simulink model "ACC_speed_change_curve_cs"  (R2016a)
settings: Solver=ode5  SolverMode=SingleTasking  StartTime=0.0  StopTime=inf  FixedStep=1/1000  RelTol=1e-3
PreLoadFcn:
  | mbxruntime.callbacks.PreLoadFcn(bdroot);
  | check_NUTS_defined;
  | 
  | assignin('base',['model_closed_' bdroot],false);addpath('../includes_ACC');
PostLoadFcn:
  | mbxruntime.callbacks.PostLoadFcn(bdroot);
InitFcn:
  | mbxruntime.callbacks.InitFcn(bdroot);
StartFcn:
  | mbxruntime.callbacks.StartFcn(bdroot);
StopFcn:
  | mbxruntime.callbacks.StopFcn(bdroot);
model workspace (MAT data in the model file):
  mbox_table : struct (value not decoded)
  model_closed = 0
  sim_status = 0
undefined symbols (not defined in the file or in its folder): DiscIntNeverNeededParam
undefined symbols (not defined in the file): SteeringColumn, SteeringWheel, WheelL0, WheelL1, WheelR0, WheelR1
libraries: simulink_extras x49, simulink x29, PreScanSimulinkLibrary x24, PreScanUsefulBlocks x2, Solver_SF x1, simulink_need_slupdate x1
(part 2 of 17)

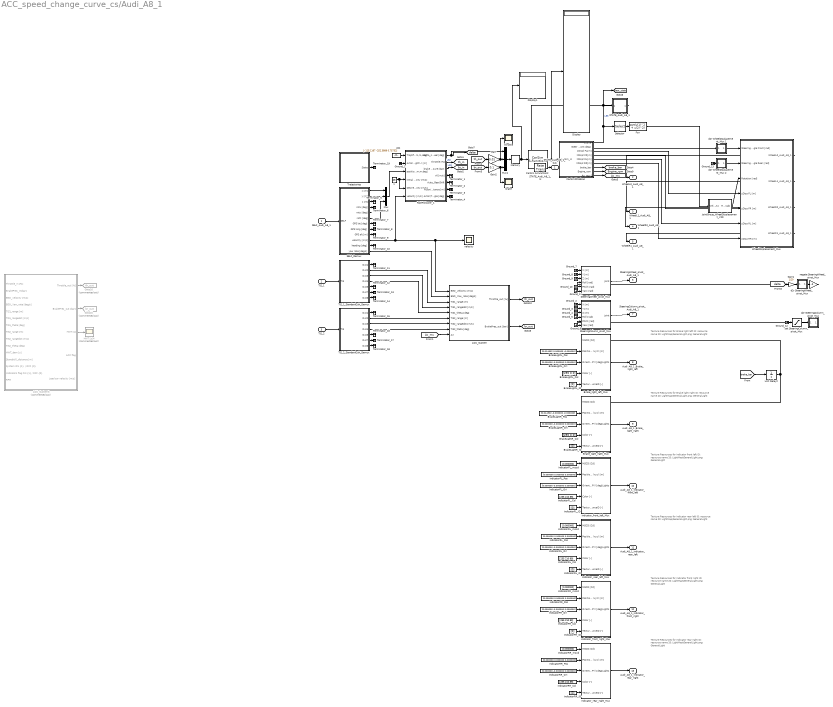
== system ACC_speed_change_curve_cs/Audi_A8_1 ==
  note: Texture Resources for Brake light left
      |
      | ID: resource name
      | 20: LightMap\GeneralLight.png: GeneralLight
  note: Texture Resources for Brake light right
      |
      | ID: resource name
      | 20: LightMap\GeneralLight.png: GeneralLight
  note: Texture Resources for Indicator front left
      |
      | ID: resource name
      | 20: LightMap\GeneralLight.png: GeneralLight
  note: Texture Resources for Indicator rear left
      |
      | ID: resource name
      | 20: LightMap\GeneralLight.png: GeneralLight
  note: Texture Resources for Indicator front right
      |
      | ID: resource name
      | 20: LightMap\GeneralLight.png: GeneralLight
  note: Texture Resources for Indicator rear right
      |
      | ID: resource name
      | 20: LightMap\GeneralLight.png: GeneralLight
  SELF_Audi_A8_1 : Inport  Tag=inport/SelfPort  OutDataTypeStr=Bus: PRESCAN_SELFSENSORDATA  PortDimensions=1  SampleTime=20/1000  BusOutputAsStruct=on
  TIS_1 : Inport  Tag=inport/TIS  Port=2  OutDataTypeStr=Bus: PRESCAN_SCANNERSENSOR_MESSAGE  PortDimensions=32  SampleTime=1/25  BusOutputAsStruct=on
  TIS_2 : Inport  Tag=inport/TIS  Port=3  OutDataTypeStr=Bus: PRESCAN_SCANNERSENSOR_MESSAGE  PortDimensions=32  SampleTime=1/25  BusOutputAsStruct=on
  ACC_System : Subsystem  mask(ACC System){J_xx=210, Rw=0.34, LaneWidth=3.5, Qfac=40.4695, BrakePressureMax=150, BrakeMax=3.5, MaxSpeed=200, drd=3, LowSpeedActv=40, TISMaxRange=[150 30], TISMaxTheta=[9 80], Tblock=1/100, TISsensor=[1/25 1/25], TISdet=[32 32], DisplaySwitch=on, DisplayFreq=25, RadarSwitch=on, RadarFreq=25}
      mask prompts: J_xx "Principal moment of inertia along longitudal (x) axis Jxx [kg*m^2]"; Rw "Tyre radius Rw [m]"; LaneWidth "Width of the lane [m]"; Qfac "Conversion factor of braking pressure into braking torque Qfac [Nm/bar]"; BrakePressureMax "Maximum brake pressure (that the controller can apply) [bar]"; BrakeMax "Maximum acceleration / deceleration, which can be applied by ACC [m/s^2]"; MaxSpeed "Maximum ACC operating velocity [km/h]"; drd "Cut-Off relatve velocity of EGO and LEAD [km/h]"; LowSpeedActv "LEAD Cut-Off Speed [km/h]"; TISMaxRange "TIS maximum range (TIS1 and TIS2) [m]"; TISMaxTheta "TIS maximum theta angle (TIS1 and TIS2) [deg]"; Tblock "Target update rate of the compilation sheet [s]"; TISsensor "TIS update rate (TIS1 and TIS2) [s]"; TISdet "TIS max. objects to detect (TIS1 and TIS2)"; DisplaySwitch "Show EGO parameters visualization"; DisplayFreq "EGO parameters visualization frequency [Hz]"; RadarSwitch "Show radar visualization"; RadarFreq "Radar frequency [Hz]"
      mask help: PreScan Experiment and Simple Dynamics model parameters
      mask init:
      | Tsensor = max([TISsensor]);
      mask Help: eval('openHelp(1131)')
      mask Callback DisplaySwitch:
      | en = get_param(gcb,'MaskEnables');
      | switch get_param(gcb, 'DisplaySwitch')
      |     case 'off'
      |         en{16} = 'off';
      |     case 'on'
      |         en{16} = 'on';
      | end
      | set_param(gcb,'MaskEnables',en);
      | clear en;
      mask Callback RadarSwitch:
      | en = get_param(gcb,'MaskEnables');
      | switch get_param(gcb, 'RadarSwitch')
      |     case 'off'
      |         en{18} = 'off';
      |     case 'on'
      |         en{18} = 'on';
      | end
      | set_param(gcb,'MaskEnables',en);
      | clear en;
  ACC_System3 : Subsystem  Commented=on  mask(ACC System){J_xx=210, Rw=0.34, LaneWidth=3.5, Qfac=40.4695, BrakePressureMax=150, MaxSpeed=200, drd=3, LowSpeedActv=40, TISMaxRange=[150 30], TISMaxTheta=[9 80], Tblock=1/100, TISsensor=[1/25 1/25], TISdet=[32 32], DisplaySwitch=on, DisplayFreq=25, RadarSwitch=on, RadarFreq=25, BrakeMax=10, BrakeRateMax=100, b=0.1, p=1, i=0.2, d=0}
      mask prompts: J_xx "Principal moment of inertia along longitudal (x) axis Jxx [kg*m^2]"; Rw "Tyre radius Rw [m]"; LaneWidth "Width of the lane [m]"; Qfac "Conversion factor of braking pressure into braking torque Qfac [Nm/bar]"; BrakePressureMax "Maximum brake pressure (that the controller can apply) [bar]"; MaxSpeed "Maximum ACC operating velocity [km/h]"; drd "Cut-Off relatve velocity of EGO and LEAD [km/h]"; LowSpeedActv "LEAD Cut-Off Speed [km/h]"; TISMaxRange "TIS maximum range (TIS1 and TIS2) [m]"; TISMaxTheta "TIS maximum theta angle (TIS1 and TIS2) [deg]"; Tblock "Target update rate of the compilation sheet [s]"; TISsensor "TIS update rate (TIS1 and TIS2) [s]"; TISdet "TIS max. objects to detect (TIS1 and TIS2)"; DisplaySwitch "Show EGO parameters visualization"; DisplayFreq "EGO parameters visualization frequency [Hz]"; RadarSwitch "Show radar visualization"; RadarFreq "Radar frequency [Hz]"; BrakeMax "Maximum acceleration / deceleration, which can be applied by ACC [m/s^2]"; BrakeRateMax "Maximum acceleration/deceleration change rate"; b "brake gain"; p "throttle p"; i "throttle i"; d "throttle d"
      mask help: PreScan Experiment and Simple Dynamics model parameters
      mask init:
      | Tsensor = max([TISsensor]);
      mask Help: eval('openHelp(1131)')
      mask Callback DisplaySwitch:
      | en = get_param(gcb,'MaskEnables');
      | switch get_param(gcb, 'DisplaySwitch')
      |     case 'off'
      |         en{16} = 'off';
      |     case 'on'
      |         en{16} = 'on';
      | end
      | set_param(gcb,'MaskEnables',en);
      | clear en;
      mask Callback RadarSwitch:
      | en = get_param(gcb,'MaskEnables');
      | switch get_param(gcb, 'RadarSwitch')
      |     case 'off'
      |         en{18} = 'off';
      |     case 'on'
      |         en{18} = 'on';
      | end
      | set_param(gcb,'MaskEnables',en);
      | clear en;
  BrakeLightL_Col : Constant  Tag=VisuLightConst  Value=[255 0 0]
  BrakeLightL_ID : Constant  Tag=VisuLightConst  Value=[0]
  BrakeLightL_Ori : Constant  Tag=VisuLightConst  Value=[0.000000 -0.000000 0.000000]
  BrakeLightL_Pos : Constant  Tag=VisuLightConst  Value=[0.014502 0.000000 -0.000000]
  BrakeLightR_Col : Constant  Tag=VisuLightConst  Value=[255 0 0]
  BrakeLightR_ID : Constant  Tag=VisuLightConst  Value=[0]
  BrakeLightR_Ori : Constant  Tag=VisuLightConst  Value=[0.000000 -0.000000 0.000000]
  BrakeLightR_Pos : Constant  Tag=VisuLightConst  Value=[0.014502 -0.000000 -0.000000]
  Brake_light_left_Mux : Subsystem  Tag=mux/ActiveLight  mask(PreScan User Interface: VisuActiveLight){}
      mask help:
      | The VisuActiveLight block provides a way for detailed animation of Light Sources, such as the indicator, brake, fog and main lights of a vehicle, or a light post.
      |
      | For more information, please click Help.
      settings: DeleteFcn=PreScanBlockDeleteFcn;
      mask Help: eval('openHelp(209)')
  Brake_light_right_Mux : Subsystem  Tag=mux/ActiveLight  mask(PreScan User Interface: VisuActiveLight){}
      mask help:
      | The VisuActiveLight block provides a way for detailed animation of Light Sources, such as the indicator, brake, fog and main lights of a vehicle, or a light post.
      |
      | For more information, please click Help.
      settings: DeleteFcn=PreScanBlockDeleteFcn;
      mask Help: eval('openHelp(209)')
  CarSim S-Function2 : Solver_SF/CarSim S-Function2  Priority=1  VehicleCode=i_i  SIMFILE=C:\Users\Public\Documents\CarSim2016Data\simfile.sim
      settings: AttributesFormatString=Vehicle Code: %<VehicleCode>
  CarSim2PreScan : Subsystem  mask(CarSim2PreScan:){z0=0, z0_ini_VRML=0.3}
      mask prompts: z0 "PreScan Actor initial COG z-position wrt GLOBAL axis system [m]"; z0_ini_VRML "z_ini_VRML [m]. Taken from : "VISUWheels_<ActorName>/conv_TransWheel.../pos_ini_Visu/z_ini_VRML" block. Use a Display Simulink block in order to visualize the value."
      mask help: This block converts the outputs coming from the CarSim block into consistent PreScan signals.
  Display : Display
  Display1 : Display
  Fcn : Fcn  Expr=sqrt(u(1)^2 + u(2)^2)
  Gain : Gain  Gain=0.01
  Gain1 : Gain  Gain=1/20
  Gain2 : Gain  Gain=0.1
  Goto15 : Goto  Commented=on  GotoTag=br_out  TagVisibility=global
  Goto16 : Goto  Commented=on  GotoTag=th_out  TagVisibility=global
  Ground_{1..13} (13 alike) : Ground
  HWT [s]4 : Scope  Commented=on
  IndicatorFL_Col : Constant  Tag=VisuLightConst  Value=[255 210 89]
  IndicatorFL_ID : Constant  Tag=VisuLightConst  Value=[0]
  IndicatorFL_Ori : Constant  Tag=VisuLightConst  Value=[0.000000 -0.000000 0.000000]
  IndicatorFL_Pos : Constant  Tag=VisuLightConst  Value=[0.000000 0.000000 0.000000]
  IndicatorFL_mscd : Constant  Tag=VisuLightConst  Value=[0.000000]
  IndicatorFR_Col : Constant  Tag=VisuLightConst  Value=[255 210 89]
  IndicatorFR_ID : Constant  Tag=VisuLightConst  Value=[0]
  IndicatorFR_Ori : Constant  Tag=VisuLightConst  Value=[0.000000 -0.000000 0.000000]
  IndicatorFR_Pos : Constant  Tag=VisuLightConst  Value=[0.000000 0.000000 0.000000]
  IndicatorFR_mscd : Constant  Tag=VisuLightConst  Value=[0.000000]
  IndicatorRL_Col : Constant  Tag=VisuLightConst  Value=[255 210 89]
  IndicatorRL_ID : Constant  Tag=VisuLightConst  Value=[0]
  IndicatorRL_Ori : Constant  Tag=VisuLightConst  Value=[0.000000 -0.000000 0.000000]
  IndicatorRL_Pos : Constant  Tag=VisuLightConst  Value=[0.000000 0.000000 0.000000]
  IndicatorRL_mscd : Constant  Tag=VisuLightConst  Value=[0.000000]
  IndicatorRR_Col : Constant  Tag=VisuLightConst  Value=[255 210 89]
  IndicatorRR_ID : Constant  Tag=VisuLightConst  Value=[0]
  IndicatorRR_Ori : Constant  Tag=VisuLightConst  Value=[0.000000 -0.000000 0.000000]
  IndicatorRR_Pos : Constant  Tag=VisuLightConst  Value=[0.000000 0.000000 0.000000]
  IndicatorRR_mscd : Constant  Tag=VisuLightConst  Value=[0.000000]
  Indicator_front_left_Mux : Subsystem  Tag=mux/ActiveLight  mask(PreScan User Interface: VisuActiveLight){}
      mask help:
      | The VisuActiveLight block provides a way for detailed animation of Light Sources, such as the indicator, brake, fog and main lights of a vehicle, or a light post.
      |
      | For more information, please click Help.
      settings: DeleteFcn=PreScanBlockDeleteFcn;
      mask Help: eval('openHelp(209)')
  Indicator_front_right_Mux : Subsystem  Tag=mux/ActiveLight  mask(PreScan User Interface: VisuActiveLight){}
      mask help:
      | The VisuActiveLight block provides a way for detailed animation of Light Sources, such as the indicator, brake, fog and main lights of a vehicle, or a light post.
      |
      | For more information, please click Help.
      settings: DeleteFcn=PreScanBlockDeleteFcn;
      mask Help: eval('openHelp(209)')
  Indicator_rear_left_Mux : Subsystem  Tag=mux/ActiveLight  mask(PreScan User Interface: VisuActiveLight){}
      mask help:
      | The VisuActiveLight block provides a way for detailed animation of Light Sources, such as the indicator, brake, fog and main lights of a vehicle, or a light post.
      |
      | For more information, please click Help.
      settings: DeleteFcn=PreScanBlockDeleteFcn;
      mask Help: eval('openHelp(209)')
  Indicator_rear_right_Mux : Subsystem  Tag=mux/ActiveLight  mask(PreScan User Interface: VisuActiveLight){}
      mask help:
      | The VisuActiveLight block provides a way for detailed animation of Light Sources, such as the indicator, brake, fog and main lights of a vehicle, or a light post.
      |
      | For more information, please click Help.
      settings: DeleteFcn=PreScanBlockDeleteFcn;
      mask Help: eval('openHelp(209)')
  JointGroup_WheelDisplacement_V2R : Subsystem  Tag=mux/Wheels  mask(PreScan Velocity to Wheel Angle Block:){TimeStep=20/1000, TireRadius=0.34000000357627869}
      mask prompts: TimeStep "Auto Assigned: Time Step [s]"; TireRadius "Tire Radius [m]"
      settings: DeleteFcn=PreScanBlockDeleteFcn;
      mask Display: disp('Velocity\nto\nWheelAngle')
  Memory : Memory
  Mux : Mux  Inputs=3
  Mux1 : Mux  Inputs=3
  PathFollower_1 : Subsystem  Tag=pathFollower  mask(PreScan Block: Path Follower){Migrate=on, FileName='Trajectory_1.mat', TunableSteeringGain=1, XShifting_wrt_COG=0}
      mask prompts: Migrate "Migrate. During migration this block will be replaced by a newer one."; FileName "Trajectory Name"; TunableSteeringGain "TunableSteeringGain [-]"; XShifting_wrt_COG "XShifting_wrt_COG [m]"
      mask help:
      | The Path Follower Model is selected in the GUI to simulate driver behavior.
      |
      | For more information, please click Help.
      mask init:
      | load(['trajectories/',eval(FileName)])
      | traject=trajectory';
      | 
      | Traj_x=traject(:,2);
      | Traj_y=traject(:,3);
      | Traj_z=traject(:,4);
      | Traj_vx=traject(:,8);
      | Traj_vy=traject(:,9);
      | Traj_vz=traject(:,10);
      mask Help: eval('openHelp(232)')
  SELF_Demux : Subsystem  Tag=demux/SelfPort  mask(PreScan Demux Block:){}
      mask help:
      | The SELF port shows (state) information of the actor itself. The outputs are position in the experiment's axis system and the GPS coordinates, and the object's absolute velocity and compass heading.
      |
      | For more information, please click Help.
      settings: DeleteFcn=PreScanBlockDeleteFcn;
      mask Help: eval('openHelp(462)')
      mask Display:
      | port_label('output',1,'x [m]')
      | port_label('output',2,'y [m]')
      | port_label('output',3,'z [m]','texmode','on')
      | port_label('output',4,'Rotx [deg]','texmode','on')
      | port_label('output',5,'Roty [deg]','texmode','on')
      | port_label('output',6,'Rotz [deg]','texmode','on')
      | port_label('output',7,'GPS lat [deg]','texmode','on')
      | port_label('output',8,'GPS long [deg]','texmode','on')
      | port_label('output',9,'GPS alt [m]','texmode','on')
      | port_label('output',10,'Velocity [m/s]')
      | port_label('output',11,'Heading [deg]')
      | port_label('output',12,'Yaw rate [deg/s]')
  STATE_Audi_A8_1 : Subsystem  Tag=mux/StatePort  Priority=0  LoadFcn=load PrescanStateActuatorData  mask(PreScan Sink Block: State){x0=-115.1167, y0=-252.3889, z0=0.55, Roll0=0, Pitch0=0, Yaw0=0.75732, TimeStep=20/1000}
      mask prompts: x0 "Ini x-position VEHICLE wrt GLOBAL axis system [m]"; y0 "Ini y-position VEHICLE wrt GLOBAL axis system [m]"; z0 "Ini z-position VEHICLE wrt GLOBAL axis system [m]"; Roll0 "Ini roll-angle BODY wrt VEHICLE axis system [deg]"; Pitch0 "Ini pitch-angle BODY wrt VEHICLE axis system [deg]"; Yaw0 "Ini yaw-angle VEHICLE wrt GLOBAL axis system [deg]"; TimeStep "Auto-Assigned: Upload Period [s]"
      mask help:
      | The Actor State contains a vector signal of size (9x1), containing the following signals:
      |
      | -  Position                  (x,y,z)                                     [m]
      | -  Velocity                  (vx,vy,vz)                               [m/s]
      | -  Angles                    (Roll, Pitch, Yaw)                   [rad]
      |
      | The Actor state is defined in the global axis system.
      | The state is superponed on the Initial position defined in the GUI.
      |
      | For more information, please click Help.
      settings: DeleteFcn=PreScanBlockDeleteFcn;
      mask Help: eval('openHelp(222)')
      mask Display: image(imread('State.png'))
  STATE_Audi_A8_1_rc : RateTransition  Tag=mux_rc/StatePort  OutPortSampleTimeOpt=Inherit
  Selector : Selector  InputPortWidth=9  IndexOptions=Index vector (dialog)  Indices=[4 5]  OutputSizes=1
  SteeringColumn_pivot_Mux : Subsystem  Tag=mux/Joint  mask(PreScan Mux Block){DisplayName=SteeringColumn}
      mask prompts: DisplayName "Display Name"
      mask help:
      | This block simulates a generic joint used for generic models. This joint can be enabled/disabled from the GUI.
      |
      | For more information, please click Help.
      settings: DeleteFcn=PreScanBlockDeleteFcn;
      mask Help: eval('openHelp(254)')
  SteeringWheel_pivot_Mux : Subsystem  Tag=mux/Joint  mask(PreScan Mux Block){DisplayName=SteeringWheel}
      mask prompts: DisplayName "Display Name"
      mask help:
      | This block simulates a generic joint used for generic models. This joint can be enabled/disabled from the GUI.
      |
      | For more information, please click Help.
      settings: DeleteFcn=PreScanBlockDeleteFcn;
      mask Help: eval('openHelp(254)')
  TIS_1_StandardCoh_Demux : Subsystem  Tag=demux/TIS/StandardCoh  TreatAsAtomicUnit=on  mask(PreScan Demux Block: TIS){MAXMESSAGES=32}
      mask prompts: MAXMESSAGES "Number of Objects"
      mask Help: eval('openHelp(449)')
      mask Display:
      | port_label('input',1,'TIS')
      | port_label('output',1,'Beam ID [-]')
      | port_label('output',2,'Range [m]')
      | port_label('output',3,'DopplerVelocity [m/s]')
      | port_label('output',4,'{\theta} [deg]','texmode','on')
      | port_label('output',5,'{\phi} [deg]','texmode','on')
      | port_label('output',6,'Target ID [-]','texmode','on')
      | port_label('output',7,'TIS Data','texmode','on')
  TIS_2_StandardCoh_Demux : Subsystem  Tag=demux/TIS/StandardCoh  TreatAsAtomicUnit=on  mask(PreScan Demux Block: TIS){MAXMESSAGES=32}
      mask prompts: MAXMESSAGES "Number of Objects"
      mask Help: eval('openHelp(449)')
      mask Display:
      | port_label('input',1,'TIS')
      | port_label('output',1,'Beam ID [-]')
      | port_label('output',2,'Range [m]')
      | port_label('output',3,'DopplerVelocity [m/s]')
      | port_label('output',4,'{\theta} [deg]','texmode','on')
      | port_label('output',5,'{\phi} [deg]','texmode','on')
      | port_label('output',6,'Target ID [-]','texmode','on')
      | port_label('output',7,'TIS Data','texmode','on')
  Terminator_{1..19} (19 alike) : Terminator
  Trajectories : Subsystem  Tag=Trajectories  mask(PreScan Source Block: Trajectories){}
      mask help:
      | The Trajectory block contains the trajectories defined in the PreScan Experiment Editor. The output of the trajectory block is the (vehicle) State.
      |
      | For more information, please click Help.
      settings: DeleteFcn=PreScanBlockDeleteFcn;
      mask Help: eval('openHelp(312)')
      mask Display: image(imread('Trajectory.png'));
  Unit Delay2 : UnitDelay  InitialCondition=1  SampleTime=-1
  V : Constant  Value=28
  WheelDisplacement_Mux : Subsystem  Tag=mux/JointGroup  mask(JointGroup){}
      mask help:
      | The JointGroup allows to control several Joints in one go, as defined for this particular model.
      | For more information, look in the PreScan manual in the section "Model Preparation Tool" -> "Joint Groups"
      |
      | For more information on the Joints simulink interface, press Help.
      mask Help: eval('openHelp(254)')
  brake : Scope
  d2r SteeringColumn_pivot_Mux : Subsystem  mask(DegreesToRadians){}
      mask help: SimulinkBlocks:simulink_extras:DegreesToRadians_MD
      mask Help: web([docroot '/simulink/ref_extras/degreestoradians.html'])
      mask Display: disp('D2R')
  d2r SteeringWheel_pivot_Mux : Subsystem  mask(DegreesToRadians){}
      mask help: SimulinkBlocks:simulink_extras:DegreesToRadians_MD
      mask Help: web([docroot '/simulink/ref_extras/degreestoradians.html'])
      mask Display: disp('D2R')
  d2r WheelDisplacement_Mux 1 : Subsystem  mask(DegreesToRadians){}
      mask help: SimulinkBlocks:simulink_extras:DegreesToRadians_MD
      mask Help: web([docroot '/simulink/ref_extras/degreestoradians.html'])
      mask Display: disp('D2R')
  d2r WheelDisplacement_Mux 2 : Subsystem  mask(DegreesToRadians){}
      mask help: SimulinkBlocks:simulink_extras:DegreesToRadians_MD
      mask Help: web([docroot '/simulink/ref_extras/degreestoradians.html'])
      mask Display: disp('D2R')
  negate SteeringWheel_pivot_Mux : Gain  Gain=-1
  pos : Constant  Tag=pos  Value=[-115.1167 -252.3889 0.75732]
  sat SteeringColumn_pivot_Mux : Saturate  UpperLimit=30  LowerLimit=-5
  throttle : Scope
  "velocity " : Scope
  STATE_Audi_A8_1_bus : Outport  Tag=outport/StatePort  OutDataTypeStr=Bus: PRESCAN_STATEACTUATORDATA  PortDimensions=1  SampleTime=20/1000
  WheelL0_Audi_A8_1 : Outport  Tag=outport/JointActuator  Port=2  OutDataTypeStr=Bus: PRESCAN_POSE_DATA  SampleTime=20/1000
  WheelL1_Audi_A8_1 : Outport  Tag=outport/JointActuator  Port=3  OutDataTypeStr=Bus: PRESCAN_POSE_DATA  SampleTime=20/1000
  WheelR0_Audi_A8_1 : Outport  Tag=outport/JointActuator  Port=4  OutDataTypeStr=Bus: PRESCAN_POSE_DATA  SampleTime=20/1000
  WheelR1_Audi_A8_1 : Outport  Tag=outport/JointActuator  Port=5  OutDataTypeStr=Bus: PRESCAN_POSE_DATA  SampleTime=20/1000
  SteeringWheel_pivot_Audi_A8_1 : Outport  Tag=outport/JointActuator  Port=6  OutDataTypeStr=Bus: PRESCAN_POSE_DATA  SampleTime=20/1000
  SteeringColumn_pivot_Audi_A8_1 : Outport  Tag=outport/JointActuator  Port=7  OutDataTypeStr=Bus: PRESCAN_POSE_DATA  SampleTime=20/1000
  Audi_A8_1_Brake_light_left : Outport  Tag=outport/BrakeLightL  Port=8  OutDataTypeStr=Bus: PRESCAN_VISULIGHTACTUATOR_DATA  SampleTime=20/1000
  Audi_A8_1_Brake_light_right : Outport  Tag=outport/BrakeLightR  Port=9  OutDataTypeStr=Bus: PRESCAN_VISULIGHTACTUATOR_DATA  SampleTime=20/1000
  Audi_A8_1_Indicator_front_left : Outport  Tag=outport/IndicatorFL  Port=10  OutDataTypeStr=Bus: PRESCAN_VISULIGHTACTUATOR_DATA  SampleTime=20/1000
  Audi_A8_1_Indicator_rear_left : Outport  Tag=outport/IndicatorRL  Port=11  OutDataTypeStr=Bus: PRESCAN_VISULIGHTACTUATOR_DATA  SampleTime=20/1000
  Audi_A8_1_Indicator_front_right : Outport  Tag=outport/IndicatorFR  Port=12  OutDataTypeStr=Bus: PRESCAN_VISULIGHTACTUATOR_DATA  SampleTime=20/1000
  Audi_A8_1_Indicator_rear_right : Outport  Tag=outport/IndicatorRR  Port=13  OutDataTypeStr=Bus: PRESCAN_VISULIGHTACTUATOR_DATA  SampleTime=20/1000
  tag scope: Ax_ms=global, Engine_rpm=global, br_in=global, br_out=global, brake_bar=global, delta=global, th_in=global, th_out=global, view_state=global
  wires:
  sat SteeringColumn_pivot_Mux/1 -> d2r SteeringColumn_pivot_Mux/1(Degrees in)
  d2r SteeringColumn_pivot_Mux/1(Radians out) -> SteeringColumn_pivot_Mux/5(Pitch [rad])
  negate SteeringWheel_pivot_Mux/1 -> SteeringWheel_pivot_Mux/4(Roll [rad])
  d2r SteeringWheel_pivot_Mux/1(Radians out) -> negate SteeringWheel_pivot_Mux/1
  [brake_bar] -> Unit Delay2/1
  Unit Delay2/1 -> Brake_light_left_Mux/1(MSCD [Cd]), Brake_light_right_Mux/1(MSCD [Cd])
  [delta] -> Gain1/1
  Gain1/1 -> d2r SteeringWheel_pivot_Mux/1(Degrees in)
  PathFollower_1/2(throttle [%]) -> [th_in]  "L82"
  PathFollower_1/3(brake pressure [bar]) -> [br_in]  "L83"
  SELF_Demux/5(roty [deg]) -> ?
  Mux/1 -> PathFollower_1/3(position x,y,Y [m,m,deg])
  SELF_Demux/1(x [m]) -> Mux/1
  SELF_Demux/2(y [m]) -> Mux/2
  SELF_Demux/6(rotz [deg]) -> Mux/3
  V/1 -> PathFollower_1/4(Initial Velocity [m/s]), PathFollower_1/5(Desired Velocity [m/s])
  d2r WheelDisplacement_Mux 1/1(Radians out) -> WheelDisplacement_Mux/1(Steering Angle Front [rad])
  d2r WheelDisplacement_Mux 2/1(Radians out) -> WheelDisplacement_Mux/2(Steering Angle Rear [rad])
  CarSim2PreScan/3(zDispl FL[m]) -> WheelDisplacement_Mux/4(zDisp FL [m])
  CarSim2PreScan/4(zDispl FR[m]) -> WheelDisplacement_Mux/5(zDisp FR [m])
  CarSim2PreScan/5(zDispl RL[m]) -> WheelDisplacement_Mux/6(zDisp RL [m])
  CarSim2PreScan/6(zDispl RR[m]) -> WheelDisplacement_Mux/7(zDisp RR [m])
  CarSim2PreScan/2(Steer Angle Front [deg]) -> d2r WheelDisplacement_Mux 1/1(Degrees in)
  CarSim2PreScan/1(STATE) -> [view_state], STATE_Audi_A8_1/1(State), Selector/1  "L86"
  Fcn/1 -> JointGroup_WheelDisplacement_V2R/1(Velocity [m/s])
  Mux1/1 -> Memory/1
  CarSim S-Function2/1 -> Display/1, CarSim2PreScan/1(CarSim_In)
  Selector/1 -> Fcn/1
  CarSim2PreScan/7(brake_bar) -> [brake_bar]
  CarSim2PreScan/8(Engine_rpm) -> [Engine_rpm]
  Memory/1 -> Display1/1, CarSim S-Function2/1
  PathFollower_1/1(delta_steerwheel [deg]) -> Mux1/1, [delta]
  [th_out] -> Gain/1
  [br_out] -> Gain2/1
  Ground_13/1 -> d2r WheelDisplacement_Mux 2/1(Degrees in)
  TIS_2_StandardCoh_Demux/3(Out3) -> ACC_System/7(TIS2_rangedot [m/s])
  SELF_Demux/12(yaw rate [deg/s]) -> ACC_System/2(EGO_Yaw_rate [deg/s])
  TIS_1_StandardCoh_Demux/2(Out2) -> ACC_System/3(TIS1_range [m])
  TIS_1_StandardCoh_Demux/3(Out3) -> ACC_System/4(TIS1_rangedot [m/s])
  TIS_1_StandardCoh_Demux/4(Out4) -> ACC_System/5(TIS1_theta [deg])
  TIS_2_StandardCoh_Demux/2(Out2) -> ACC_System/6(TIS2_range [m])
  TIS_2_StandardCoh_Demux/4(Out4) -> ACC_System/8(TIS2_theta [deg])
  SELF_Demux/10(velocity [m/s]) -> ACC_System/1(EGO_velocity [m/s]), "velocity "/1, PathFollower_1/6(velocity [m/s])
  CarSim2PreScan/9(Ax_ms-1) -> [Ax_ms]
  Gain/1 -> throttle/1, Mux1/2
  Gain2/1 -> brake/1, Mux1/3
  ACC_System3/1(Throttle_out [%]) -> Goto16/1
  ACC_System3/2(BrakePres_out [bar]) -> Goto15/1
  ACC_System3/3(HWT [s]) -> HWT [s]4/1
  ACC_System/1(Throttle_out [%]) -> [th_out]
  ACC_System/2(BrakePres_out [bar]) -> [br_out]
  [Ax_ms] -> ACC_System/9(AX)
  STATE_Audi_A8_1_rc/1 -> STATE_Audi_A8_1_bus/1
  STATE_Audi_A8_1/1(StateBus) -> STATE_Audi_A8_1_rc/1
  SELF_Audi_A8_1/1 -> SELF_Demux/1(SELF)
  TIS_1/1 -> TIS_1_StandardCoh_Demux/1(TIS)
  TIS_2/1 -> TIS_2_StandardCoh_Demux/1(TIS)
  WheelDisplacement_Mux/1(WheelL0_Audi_A8_1) -> WheelL0_Audi_A8_1/1
  WheelDisplacement_Mux/2(WheelL1_Audi_A8_1) -> WheelL1_Audi_A8_1/1
  WheelDisplacement_Mux/3(WheelR0_Audi_A8_1) -> WheelR0_Audi_A8_1/1
  WheelDisplacement_Mux/4(WheelR1_Audi_A8_1) -> WheelR1_Audi_A8_1/1
  JointGroup_WheelDisplacement_V2R/1(Rotation [rad]) -> WheelDisplacement_Mux/3(Rotation [rad])
  SteeringWheel_pivot_Mux/1(Joint) -> SteeringWheel_pivot_Audi_A8_1/1
  SteeringColumn_pivot_Mux/1(Joint) -> SteeringColumn_pivot_Audi_A8_1/1
  Brake_light_left_Mux/1(Lights) -> Audi_A8_1_Brake_light_left/1
  BrakeLightL_Pos/1 -> Brake_light_left_Mux/2(Position (xyz) [m])
  BrakeLightL_Ori/1 -> Brake_light_left_Mux/3(Orientation (RPY) [deg])
  BrakeLightL_Col/1 -> Brake_light_left_Mux/4(Color [-])
  BrakeLightL_ID/1 -> Brake_light_left_Mux/5(TextureResourceID [-])
  Brake_light_right_Mux/1(Lights) -> Audi_A8_1_Brake_light_right/1
  BrakeLightR_Pos/1 -> Brake_light_right_Mux/2(Position (xyz) [m])
  BrakeLightR_Ori/1 -> Brake_light_right_Mux/3(Orientation (RPY) [deg])
  BrakeLightR_Col/1 -> Brake_light_right_Mux/4(Color [-])
  BrakeLightR_ID/1 -> Brake_light_right_Mux/5(TextureResourceID [-])
  Indicator_front_left_Mux/1(Lights) -> Audi_A8_1_Indicator_front_left/1
  IndicatorFL_mscd/1 -> Indicator_front_left_Mux/1(MSCD [Cd])
  IndicatorFL_Pos/1 -> Indicator_front_left_Mux/2(Position (xyz) [m])
  IndicatorFL_Ori/1 -> Indicator_front_left_Mux/3(Orientation (RPY) [deg])
  IndicatorFL_Col/1 -> Indicator_front_left_Mux/4(Color [-])
  IndicatorFL_ID/1 -> Indicator_front_left_Mux/5(TextureResourceID [-])
  Indicator_rear_left_Mux/1(Lights) -> Audi_A8_1_Indicator_rear_left/1
  IndicatorRL_mscd/1 -> Indicator_rear_left_Mux/1(MSCD [Cd])
  IndicatorRL_Pos/1 -> Indicator_rear_left_Mux/2(Position (xyz) [m])
  IndicatorRL_Ori/1 -> Indicator_rear_left_Mux/3(Orientation (RPY) [deg])
  IndicatorRL_Col/1 -> Indicator_rear_left_Mux/4(Color [-])
  IndicatorRL_ID/1 -> Indicator_rear_left_Mux/5(TextureResourceID [-])
  Indicator_front_right_Mux/1(Lights) -> Audi_A8_1_Indicator_front_right/1
  IndicatorFR_mscd/1 -> Indicator_front_right_Mux/1(MSCD [Cd])
  IndicatorFR_Pos/1 -> Indicator_front_right_Mux/2(Position (xyz) [m])
  IndicatorFR_Ori/1 -> Indicator_front_right_Mux/3(Orientation (RPY) [deg])
  IndicatorFR_Col/1 -> Indicator_front_right_Mux/4(Color [-])
  IndicatorFR_ID/1 -> Indicator_front_right_Mux/5(TextureResourceID [-])
  Indicator_rear_right_Mux/1(Lights) -> Audi_A8_1_Indicator_rear_right/1
  IndicatorRR_mscd/1 -> Indicator_rear_right_Mux/1(MSCD [Cd])
  IndicatorRR_Pos/1 -> Indicator_rear_right_Mux/2(Position (xyz) [m])
  IndicatorRR_Ori/1 -> Indicator_rear_right_Mux/3(Orientation (RPY) [deg])
  IndicatorRR_Col/1 -> Indicator_rear_right_Mux/4(Color [-])
  IndicatorRR_ID/1 -> Indicator_rear_right_Mux/5(TextureResourceID [-])
  pos/1 -> PathFollower_1/1(TrajOffset_x,y,Y [m,m,deg])
  Ground_1/1 -> PathFollower_1/2(ActorOffset_Left(+) / Right(-) [m])
  PathFollower_1/4(v0 [m/s]) -> Terminator_1/1
  PathFollower_1/5(Auto_GearShift) -> Terminator_2/1
  PathFollower_1/6(Actor/Traj_distance [m]) -> Terminator_3/1
  PathFollower_1/7(Actor/Traj_angle [deg]) -> Terminator_4/1
  SELF_Demux/3(z [m]) -> Terminator_5/1
  SELF_Demux/4(rotx [deg]) -> Terminator_6/1
  SELF_Demux/7(GPS lat [deg]) -> Terminator_7/1
  SELF_Demux/8(GPS long [deg]) -> Terminator_8/1
  SELF_Demux/9(GPS alt [m]) -> Terminator_9/1
  SELF_Demux/11(heading [deg]) -> Terminator_10/1
  Ground_2/1 -> SteeringColumn_pivot_Mux/1(X [m])
  Ground_3/1 -> SteeringColumn_pivot_Mux/2(Y [m])
  Ground_4/1 -> SteeringColumn_pivot_Mux/3(Z [m])
  Ground_5/1 -> SteeringColumn_pivot_Mux/4(Roll [rad])
  Ground_6/1 -> SteeringColumn_pivot_Mux/6(Yaw [rad])
  Ground_7/1 -> SteeringWheel_pivot_Mux/1(X [m])
  Ground_8/1 -> SteeringWheel_pivot_Mux/2(Y [m])
  Ground_9/1 -> SteeringWheel_pivot_Mux/3(Z [m])
  Ground_10/1 -> SteeringWheel_pivot_Mux/5(Pitch [rad])
  Ground_11/1 -> SteeringWheel_pivot_Mux/6(Yaw [rad])
  TIS_1_StandardCoh_Demux/1(Out1) -> Terminator_11/1
  TIS_1_StandardCoh_Demux/5(Out5) -> Terminator_12/1
  TIS_1_StandardCoh_Demux/6(Out7) -> Terminator_13/1
  TIS_1_StandardCoh_Demux/7(Out6) -> Terminator_14/1
  TIS_2_StandardCoh_Demux/1(Out1) -> Terminator_15/1
  TIS_2_StandardCoh_Demux/5(Out5) -> Terminator_16/1
  TIS_2_StandardCoh_Demux/6(Out7) -> Terminator_17/1
  TIS_2_StandardCoh_Demux/7(Out6) -> Terminator_18/1
  Trajectories/1(State) -> Terminator_19/1
  Ground_12/1 -> sat SteeringColumn_pivot_Mux/1

== system ACC_speed_change_curve_cs/Audi_A8_1_Brake_light_left ==
  Audi_A8_1_Brake_light_left : Inport  Tag=inport/BrakeLightL  OutDataTypeStr=Bus: PRESCAN_VISULIGHTACTUATOR_DATA  SampleTime=20/1000  BusOutputAsStruct=on
  Actuator : S-Function  FunctionName=sfun_VisuLightActuator  Parameters=mbxruntime.parameters.convert(UniqueID), mbxruntime.parameters.convert(LightName), mbxruntime.parameters.convert(PivotName), mbxruntime.parameters.convert(TextureResources), mbxruntime.parameters.convert(ColorsObjectName), mbxruntime.parameters.convert(MeshOnColor), mbxruntime.parameters.convert(MeshOffColor),tabledata, TimeStep  SFunctionDeploymentMode=off  EnableBusSupport=off  mask(PreScan Sink Block: VisuActiveLight){UniqueID=13, LightName=Audi_A8_1.LightActuator_0_BrakeLightRL_ActiveLight, PivotName=Audi_A8_1.BrakeLightL_pivot, TextureResources={ '20' 'LightMap\GeneralLight.png'}, ColorsObjectName=Audi_A8_1.BrakeLightRL, MeshOnColor=[255    0    0  255  255    0    0  255  102  102  102  255  510    0    0  255], MeshOffColor=[255    0    0  255  255    0    0  255  102  102  102  255    0    0    0  255], TimeStep=20/1000}
      mask prompts: UniqueID "Parent Unique Identifier"; LightName "Light"; PivotName "Pivot"; TextureResources "Texture Resources"; ColorsObjectName "Light Fixture Color Object"; MeshOnColor "Light Fixture On Color"; MeshOffColor "Light Fixture Off Color"; TimeStep "Simulink time step"
      mask help:
      | The VisuActiveLight block provides a way for detailed animation of Light Sources, such as the indicator, brake, fog and main lights of a vehicle, or a light post.
      |
      | For more information, please click Help.
      mask init:
      | [tabledata] = mbxruntime.parameters.table(UniqueID,LightName,PivotName,TextureResources,ColorsObjectName,MeshOnColor,MeshOffColor);
      mask Help: eval('openHelp(209)')
      mask Display: image(imread('HeadLight.png'))
  wires:
  Audi_A8_1_Brake_light_left/1 -> Actuator/1

== system ACC_speed_change_curve_cs/Audi_A8_1_Brake_light_right ==
  Audi_A8_1_Brake_light_right : Inport  Tag=inport/BrakeLightR  OutDataTypeStr=Bus: PRESCAN_VISULIGHTACTUATOR_DATA  SampleTime=20/1000  BusOutputAsStruct=on
  Actuator : S-Function  FunctionName=sfun_VisuLightActuator  Parameters=mbxruntime.parameters.convert(UniqueID), mbxruntime.parameters.convert(LightName), mbxruntime.parameters.convert(PivotName), mbxruntime.parameters.convert(TextureResources), mbxruntime.parameters.convert(ColorsObjectName), mbxruntime.parameters.convert(MeshOnColor), mbxruntime.parameters.convert(MeshOffColor),tabledata, TimeStep  SFunctionDeploymentMode=off  EnableBusSupport=off  mask(PreScan Sink Block: VisuActiveLight){UniqueID=13, LightName=Audi_A8_1.LightActuator_1_BrakeLightRR_ActiveLight, PivotName=Audi_A8_1.BrakeLightR_pivot, TextureResources={ '20' 'LightMap\GeneralLight.png'}, ColorsObjectName=Audi_A8_1.BrakeLightRR, MeshOnColor=[255    0    0  255  255    0    0  255  102  102  102  255  510    0    0  255], MeshOffColor=[255    0    0  255  255    0    0  255  102  102  102  255    0    0    0  255], TimeStep=20/1000}
      mask prompts: UniqueID "Parent Unique Identifier"; LightName "Light"; PivotName "Pivot"; TextureResources "Texture Resources"; ColorsObjectName "Light Fixture Color Object"; MeshOnColor "Light Fixture On Color"; MeshOffColor "Light Fixture Off Color"; TimeStep "Simulink time step"
      mask help:
      | The VisuActiveLight block provides a way for detailed animation of Light Sources, such as the indicator, brake, fog and main lights of a vehicle, or a light post.
      |
      | For more information, please click Help.
      mask init:
      | [tabledata] = mbxruntime.parameters.table(UniqueID,LightName,PivotName,TextureResources,ColorsObjectName,MeshOnColor,MeshOffColor);
      mask Help: eval('openHelp(209)')
      mask Display: image(imread('HeadLight.png'))
  wires:
  Audi_A8_1_Brake_light_right/1 -> Actuator/1

== system ACC_speed_change_curve_cs/Audi_A8_1_Indicator_front_left ==
  Audi_A8_1_Indicator_front_left : Inport  Tag=inport/IndicatorFL  OutDataTypeStr=Bus: PRESCAN_VISULIGHTACTUATOR_DATA  SampleTime=20/1000  BusOutputAsStruct=on
  Actuator : S-Function  FunctionName=sfun_VisuLightActuator  Parameters=mbxruntime.parameters.convert(UniqueID), mbxruntime.parameters.convert(LightName), mbxruntime.parameters.convert(PivotName), mbxruntime.parameters.convert(TextureResources), mbxruntime.parameters.convert(ColorsObjectName), mbxruntime.parameters.convert(MeshOnColor), mbxruntime.parameters.convert(MeshOffColor),tabledata, TimeStep  SFunctionDeploymentMode=off  EnableBusSupport=off  mask(PreScan Sink Block: VisuActiveLight){UniqueID=13, LightName=Audi_A8_1.LightActuator_6_IndicatorFL_ActiveLight, PivotName=Audi_A8_1.IndicatorFL_pivot, TextureResources={ '20' 'LightMap\GeneralLight.png'}, ColorsObjectName=Audi_A8_1.IndicatorFL, MeshOnColor=[255  165    0    0  255  165    0    0  102  102  102  255  510  420  178  255], MeshOffColor=[255  165    0    0  255  165    0    0  102  102  102  255    0    0    0  255], TimeStep=20/1000}
      mask prompts: UniqueID "Parent Unique Identifier"; LightName "Light"; PivotName "Pivot"; TextureResources "Texture Resources"; ColorsObjectName "Light Fixture Color Object"; MeshOnColor "Light Fixture On Color"; MeshOffColor "Light Fixture Off Color"; TimeStep "Simulink time step"
      mask help:
      | The VisuActiveLight block provides a way for detailed animation of Light Sources, such as the indicator, brake, fog and main lights of a vehicle, or a light post.
      |
      | For more information, please click Help.
      mask init:
      | [tabledata] = mbxruntime.parameters.table(UniqueID,LightName,PivotName,TextureResources,ColorsObjectName,MeshOnColor,MeshOffColor);
      mask Help: eval('openHelp(209)')
      mask Display: image(imread('HeadLight.png'))
  wires:
  Audi_A8_1_Indicator_front_left/1 -> Actuator/1

== system ACC_speed_change_curve_cs/Audi_A8_1_Indicator_front_right ==
  Audi_A8_1_Indicator_front_right : Inport  Tag=inport/IndicatorFR  OutDataTypeStr=Bus: PRESCAN_VISULIGHTACTUATOR_DATA  SampleTime=20/1000  BusOutputAsStruct=on
  Actuator : S-Function  FunctionName=sfun_VisuLightActuator  Parameters=mbxruntime.parameters.convert(UniqueID), mbxruntime.parameters.convert(LightName), mbxruntime.parameters.convert(PivotName), mbxruntime.parameters.convert(TextureResources), mbxruntime.parameters.convert(ColorsObjectName), mbxruntime.parameters.convert(MeshOnColor), mbxruntime.parameters.convert(MeshOffColor),tabledata, TimeStep  SFunctionDeploymentMode=off  EnableBusSupport=off  mask(PreScan Sink Block: VisuActiveLight){UniqueID=13, LightName=Audi_A8_1.LightActuator_8_IndicatorFR_ActiveLight, PivotName=Audi_A8_1.IndicatorFR_pivot, TextureResources={ '20' 'LightMap\GeneralLight.png'}, ColorsObjectName=Audi_A8_1.IndicatorFR, MeshOnColor=[255  165    0    0  255  165    0    0  102  102  102  255  510  420  178  255], MeshOffColor=[255  165    0    0  255  165    0    0  102  102  102  255    0    0    0  255], TimeStep=20/1000}
      mask prompts: UniqueID "Parent Unique Identifier"; LightName "Light"; PivotName "Pivot"; TextureResources "Texture Resources"; ColorsObjectName "Light Fixture Color Object"; MeshOnColor "Light Fixture On Color"; MeshOffColor "Light Fixture Off Color"; TimeStep "Simulink time step"
      mask help:
      | The VisuActiveLight block provides a way for detailed animation of Light Sources, such as the indicator, brake, fog and main lights of a vehicle, or a light post.
      |
      | For more information, please click Help.
      mask init:
      | [tabledata] = mbxruntime.parameters.table(UniqueID,LightName,PivotName,TextureResources,ColorsObjectName,MeshOnColor,MeshOffColor);
      mask Help: eval('openHelp(209)')
      mask Display: image(imread('HeadLight.png'))
  wires:
  Audi_A8_1_Indicator_front_right/1 -> Actuator/1

== system ACC_speed_change_curve_cs/Audi_A8_1_Indicator_rear_left ==
  Audi_A8_1_Indicator_rear_left : Inport  Tag=inport/IndicatorRL  OutDataTypeStr=Bus: PRESCAN_VISULIGHTACTUATOR_DATA  SampleTime=20/1000  BusOutputAsStruct=on
  Actuator : S-Function  FunctionName=sfun_VisuLightActuator  Parameters=mbxruntime.parameters.convert(UniqueID), mbxruntime.parameters.convert(LightName), mbxruntime.parameters.convert(PivotName), mbxruntime.parameters.convert(TextureResources), mbxruntime.parameters.convert(ColorsObjectName), mbxruntime.parameters.convert(MeshOnColor), mbxruntime.parameters.convert(MeshOffColor),tabledata, TimeStep  SFunctionDeploymentMode=off  EnableBusSupport=off  mask(PreScan Sink Block: VisuActiveLight){UniqueID=13, LightName=Audi_A8_1.LightActuator_7_IndicatorRL_ActiveLight, PivotName=Audi_A8_1.IndicatorRL_pivot, TextureResources={ '20' 'LightMap\GeneralLight.png'}, ColorsObjectName=Audi_A8_1.IndicatorRL, MeshOnColor=[255  165    0    0  255  165    0    0  102  102  102  255  510  420  178  255], MeshOffColor=[255  165    0    0  255  165    0    0  102  102  102  255    0    0    0  255], TimeStep=20/1000}
      mask prompts: UniqueID "Parent Unique Identifier"; LightName "Light"; PivotName "Pivot"; TextureResources "Texture Resources"; ColorsObjectName "Light Fixture Color Object"; MeshOnColor "Light Fixture On Color"; MeshOffColor "Light Fixture Off Color"; TimeStep "Simulink time step"
      mask help:
      | The VisuActiveLight block provides a way for detailed animation of Light Sources, such as the indicator, brake, fog and main lights of a vehicle, or a light post.
      |
      | For more information, please click Help.
      mask init:
      | [tabledata] = mbxruntime.parameters.table(UniqueID,LightName,PivotName,TextureResources,ColorsObjectName,MeshOnColor,MeshOffColor);
      mask Help: eval('openHelp(209)')
      mask Display: image(imread('HeadLight.png'))
  wires:
  Audi_A8_1_Indicator_rear_left/1 -> Actuator/1

== system ACC_speed_change_curve_cs/Audi_A8_1_Indicator_rear_right ==
  Audi_A8_1_Indicator_rear_right : Inport  Tag=inport/IndicatorRR  OutDataTypeStr=Bus: PRESCAN_VISULIGHTACTUATOR_DATA  SampleTime=20/1000  BusOutputAsStruct=on
  Actuator : S-Function  FunctionName=sfun_VisuLightActuator  Parameters=mbxruntime.parameters.convert(UniqueID), mbxruntime.parameters.convert(LightName), mbxruntime.parameters.convert(PivotName), mbxruntime.parameters.convert(TextureResources), mbxruntime.parameters.convert(ColorsObjectName), mbxruntime.parameters.convert(MeshOnColor), mbxruntime.parameters.convert(MeshOffColor),tabledata, TimeStep  SFunctionDeploymentMode=off  EnableBusSupport=off  mask(PreScan Sink Block: VisuActiveLight){UniqueID=13, LightName=Audi_A8_1.LightActuator_9_IndicatorRR_ActiveLight, PivotName=Audi_A8_1.IndicatorRR_pivot, TextureResources={ '20' 'LightMap\GeneralLight.png'}, ColorsObjectName=Audi_A8_1.IndicatorRR, MeshOnColor=[255  165    0    0  255  165    0    0  102  102  102  255  510  420  178  255], MeshOffColor=[255  165    0    0  255  165    0    0  102  102  102  255    0    0    0  255], TimeStep=20/1000}
      mask prompts: UniqueID "Parent Unique Identifier"; LightName "Light"; PivotName "Pivot"; TextureResources "Texture Resources"; ColorsObjectName "Light Fixture Color Object"; MeshOnColor "Light Fixture On Color"; MeshOffColor "Light Fixture Off Color"; TimeStep "Simulink time step"
      mask help:
      | The VisuActiveLight block provides a way for detailed animation of Light Sources, such as the indicator, brake, fog and main lights of a vehicle, or a light post.
      |
      | For more information, please click Help.
      mask init:
      | [tabledata] = mbxruntime.parameters.table(UniqueID,LightName,PivotName,TextureResources,ColorsObjectName,MeshOnColor,MeshOffColor);
      mask Help: eval('openHelp(209)')
      mask Display: image(imread('HeadLight.png'))
  wires:
  Audi_A8_1_Indicator_rear_right/1 -> Actuator/1
